simulink model "NEW3"  (Simulink 7.4)
settings: Solver=FixedStepDiscrete  SolverMode=SingleTasking  StartTime=0.0  StopTime=inf  FixedStep=1/8000  RelTol=1e-3
undefined symbols (not defined in the file or in its folder): bit
libraries: c6713dsklib x2, dspxfrm3 x2, idelinklib_tgtpref x1
settings Model: Creator=jagi20  LastModifiedBy=Chris
settings SolverCC: PositivePriorityOrder=on
settings DataIOCC: SaveOutput=off  SaveTime=off
settings HardwareCC: ProdBitPerLong=40  ProdIntDivRoundTo=Zero  ProdEndianess=LittleEndian  ProdHWDeviceType=Texas Instruments->C6000
settings RTWCC: SystemTargetFile=ccslink_grt.tlc  GenCodeOnly=on  GenerateMakefile=off  TemplateMakefile=none  Description=Embedded IDE Link (for use with Texas Instruments(TM) Code Composer Studio(TM)) GRT code generation  ProcessScript=ccslink_grt_make_rtw_hook
settings GRTTgtLinkCCS: TargetFcnLib=ansi_tfl_table_tmw.mat  TargetFunctionLibrary=ANSI_C  UtilityFuncGeneration=Auto  ERTMultiwordTypeDef=System defined  ERTMultiwordLength=256  MultiwordLength=2048  GenerateFullHeader=on  GenerateSampleERTMain=off  GenerateTestInterfaces=off  IsPILTarget=off  ModelReferenceCompliant=on  ParMdlRefBuildCompliant=off  CompOptLevelCompliant=off  IncludeMdlTerminateFcn=on  GeneratePreprocessorConditionals=Disable all  CombineOutputUpdateFcns=off  SuppressErrorStatus=off  ERTFirstTimeCompliant=off  IncludeFileDelimiter=Auto  ERTCustomFileBanners=off  SupportAbsoluteTime=on  LogVarNameModifier=rt_  MatFileLogging=off  MultiInstanceERTCode=off  SupportNonFinite=on  SupportComplex=on  PurelyIntegerCode=off  SupportContinuousTime=on  SupportNonInlinedSFcns=on  SupportVariableSizeSignals=off  EnableShiftOperators=on  ParenthesesLevel=Nominal  PortableWordSizes=off  ModelStepFunctionPrototypeControlCompliant=off  CPPClassGenCompliant=off  AutosarCompliant=off  GenerateASAP2=off  ExtMode=off  ExtModeTransport=0  ExtModeStaticAlloc=off  ExtModeStaticAllocSize=1000000  ExtModeTesting=off  ExtModeMexFile=ext_comm  ExtModeIntrfLevel=Level1  RTWCAPISignals=off  RTWCAPIParams=off  RTWCAPIStates=off  exportCCSObj=on  ccsObjName=CCS_Obj  exportIDEObj=on  ideObjName=CCS_Obj  oldideObjName=CCS_Obj  ideObjTimeout=10  oldideObjTimeout=10  ideObjBuildTimeout=1000  oldideObjBuildTimeout=1000  ProfileGenCode=off  profileBy=Tasks  ProfileNumSamples=100  InlineDSPBlks=off  projectOptions=Custom  debugCompilerOptions="-g -d\"_DEBUG\""  releaseCompilerOptions=-o2  customCompilerOptions=o2 -q  compilerOptionsStr=o2 -q  getCompilerOptions=off  getLinkerOptions=off  systemStackSize=8192  buildAction=Build_and_execute  overrunNotificationMethod=None  overrunNotificationFcn=myfunction  oldoverrunNotificationFcn=myfunction  DiagnosticActions=warning

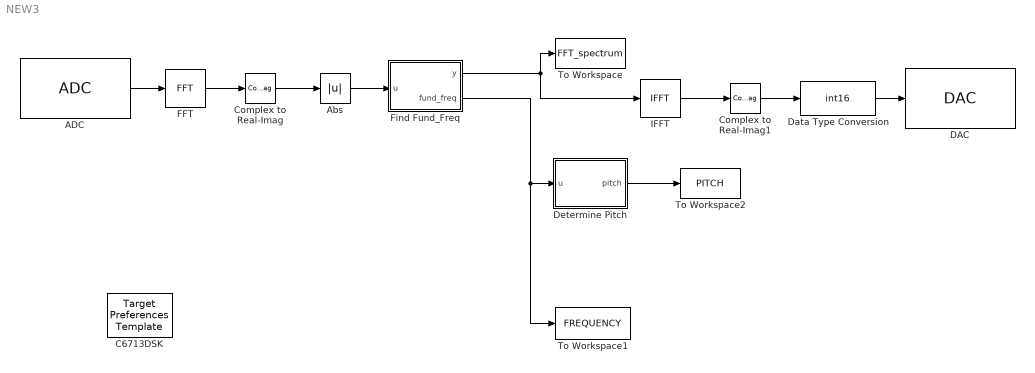
== system NEW3 ==
  ADC : c6713dsklib/ADC  ADCsource=Mic In  MicGain=off  Stereo=off  SampleRate=8 kHz  CodecDataFormat=16-bit  OutputDataType=Single  Scaling=Normalize  SourceGain=0.0  FrameSize=1  inheritSampleTime=off
  Abs : Abs  OutDataTypeMode=int16  OutDataType=fixdt(1, 16)  OutScaling=2^0  OutDataTypeStr=int16
  C6713DSK : idelinklib_tgtpref/Target Preferences Template  Tag=ccslinktgtpref  SystemSampleTime=-1
  Complex to Real-Imag : ComplexToRealImag  Output=Real
  Complex to Real-Imag1 : ComplexToRealImag  Output=Real
  DAC : c6713dsklib/DAC  CodecDataFormat=16-bit  SampleRate=8 kHz  Scaling=Normalize  DacAtten=0.0  OverflowMode=Wrap
  Data Type Conversion : DataTypeConversion  OutDataTypeMode=int16  OutDataType=fixdt(1, 16)  OutScaling=2^0  OutDataTypeStr=int16
  Determine Pitch : Stateflow chart
  FFT : dspxfrm3/FFT  DialogController=dspDDGCreate  DialogControllerArgs=DataTag1  CompMethod=Table lookup  TableOpt=NEW  TableOptActive=Speed  BitRevOrder=off  InheritFFTLength=off  FFTLength=64  SkipNorm=off  roundingMode=Floor  overflowMode=off
  Find Fund_Freq : Stateflow chart
  IFFT : dspxfrm3/IFFT  DialogController=dspDDGCreate  DialogControllerArgs=DataTag2  CompMethod=Table lookup  TableOpt=NEW  TableOptActive=Speed  BitRevOrder=off  cs_in=off  SkipNorm=on  InheritFFTLength=on  FFTLength=64  mode=Complex  outSamplingMode=Sample based  roundingMode=Floor  overflowMode=off
  To Workspace : ToWorkspace  VariableName=FFT_spectrum  SampleTime=-1  SaveFormat=Array
  To Workspace1 : ToWorkspace  VariableName=FREQUENCY  SampleTime=-1  SaveFormat=Array
  To Workspace2 : ToWorkspace  VariableName=PITCH  SampleTime=-1  SaveFormat=Array
  wires:
  Abs/1 -> Find Fund_Freq/1(u)
  Find Fund_Freq/1(y) -> To Workspace/1, IFFT/1
  Find Fund_Freq/2(fund_freq) -> To Workspace1/1, Determine Pitch/1(u)
  FFT/1 -> Complex to Real-Imag/1
  Complex to Real-Imag/1 -> Abs/1
  Determine Pitch/1(pitch) -> To Workspace2/1
  Complex to Real-Imag1/1 -> Data Type Conversion/1
  IFFT/1 -> Complex to Real-Imag1/1
  ADC/1 -> FFT/1
  Data Type Conversion/1 -> DAC/1

== matlab function Determine Pitch ==
  data: u input double; pitch output double
function pitch = fcn(u)
%#eml

pitch = double(0.0); %initialize pitch value

% AMERICAN STANDARD PITCHES (all in Hz)
% A = 220;
% A1 = 233; % A sharp
% B = 247;
% C = 262; % 'middle C'
% C1 = 277;
% D = 294;
% D1 = 311;
% E = 330;
% F = 349;
% F1 = 370;
% G = 392;
% G1 = 415;

f = round(u); %round to nearest integer

if (f==0) %THIS IS AN ERROR!
    pitch = 9.99999999999999;
elseif (f ~=0)

i=0; %index for iterations of the following loop
while ((f < 212) || (f > 425))
    if f <= 210 %lower octave
        f = 2*f;
        i = i+1;
    elseif (f > 430) 
        f = 0.5*f;
        i = i+1;
    elseif (i > 9999) %prevent inf loop
        break;
    end
end

f = round(f); %make sure it's an integer (again)

if ((212 <= f) && (f <= 226)) 
    pitch = double('A') + .0001*double('0');
elseif ((227 <= f) && (f <= 240)) 
    pitch = double('A') + .0001*double('1');
elseif ((241 <= f) && (f <= 254)) 
    pitch = double('B') + .0001*double('0');
elseif ((255 <= f) && (f <= 269)) 
    pitch = double('C') + .0001*double('0');
elseif ((270 <= f) && (f <= 285)) 
    pitch = double('C') + .0001*double('1');
elseif ((286 <= f) && (f <= 302)) 
    pitch = double('D') + .0001*double('0');
elseif ((303 <= f) && (f <= 320)) 
    pitch = double('D') + .0001*double('1');
elseif ((321 <= f) && (f <= 339)) 
    pitch = double('E') + .0001*double('0');
elseif ((340 <= f) && (f <= 359))
    pitch = double('F') + .0001*double('0');
elseif ((360 <= f) && (f <= 381))
    pitch = double('F') + .0001*double('1');
elseif ((382 <= f) && (f <= 403)) 
    pitch = double('G') + .0001*double('0');
elseif ((404 <= f) && (f <= 425))
    pitch = double('G') + .0001*double('1');
end

end

== matlab function Find Fund_Freq ==
  data: u input double; y output double; fund_freq output int16
function [y,fund_freq] = fcn(u)
%#eml
q = u(:,1);
y = q;

value = max(q);
a = int16(find(q==value,1) -1);
fund_freq = a(1,1); %a scalar
